simulink model "HW5_2_A"  (R2016a)
settings: Solver=VariableStepAuto  StartTime=0.0  StopTime=50  RelTol=1e-3
settings Model: Creator=Teng-Hu  LastModifiedBy=Teng-Hu
settings GRTTargetCC: GeneratePreprocessorConditionals=Use local settings

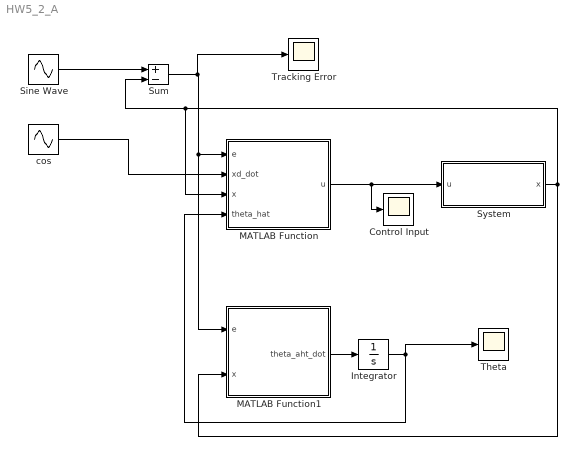
== system HW5_2_A ==
  Control Input : Scope
  Integrator : Integrator  InitialCondition=[1 ;1]
  MATLAB Function : MATLAB Function  TreatAsAtomicUnit=on
  MATLAB Function1 : MATLAB Function  TreatAsAtomicUnit=on
  Sine Wave : Sin  SampleTime=0
  Sum : Sum  Inputs=+-
  System : Subsystem
  Theta : Scope
  Tracking Error : Scope
  "cos " : Sin  Phase=pi/2  SampleTime=0
  wires:
  MATLAB Function/1(u) -> Control Input/1, System/1(u)
  Sine Wave/1 -> Sum/1
  System/1(x) -> MATLAB Function1/2(x), MATLAB Function/3(x), Sum/2
  Sum/1 -> Tracking Error/1, MATLAB Function1/1(e), MATLAB Function/1(e)
  "cos "/1 -> MATLAB Function/2(xd_dot)
  MATLAB Function1/1(theta_aht_dot) -> Integrator/1
  Integrator/1 -> MATLAB Function/4(theta_hat), Theta/1

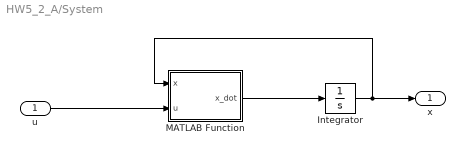
== system HW5_2_A/System ==
  u : Inport
  Integrator : Integrator  InitialCondition=1
  MATLAB Function : MATLAB Function  TreatAsAtomicUnit=on
  x : Outport
  wires:
  MATLAB Function/1(x_dot) -> Integrator/1
  Integrator/1 -> MATLAB Function/1(x), x/1
  u/1 -> MATLAB Function/2(u)

== matlab function HW5_2_A/MATLAB Function ==
  data: e input; u output; xd_dot input; x input; theta_hat input
function u = fcn(e,xd_dot,x, theta_hat)
%#codegen
k=5;
Y_T=[x;cos(x)]
u = xd_dot-Y_T'*theta_hat+k*e;

== matlab function HW5_2_A/System/MATLAB Function ==
  data: x input; u input; x_dot output
function x_dot = fcn(x,u)
%#codegen

x_dot = 2*x+5*cos(x)+u;

== matlab function HW5_2_A/MATLAB Function1 ==
  data: e input; theta_aht_dot output; x input
function theta_aht_dot      = fcn(e,x)
%#codegen
gamma=5;
Y_T=[x;cos(x)];
theta_aht_dot = -gamma*Y_T*e;
